simulink model "Multimedia_IP_traffic"  (R2021a)
settings: Solver=VariableStepAuto  StartTime=0.0  StopTime=10.0  RelTol=1e-3
settings Model: Creator=Ebenezer Sarpong  LastModifiedBy=Ebenezer Sarpong

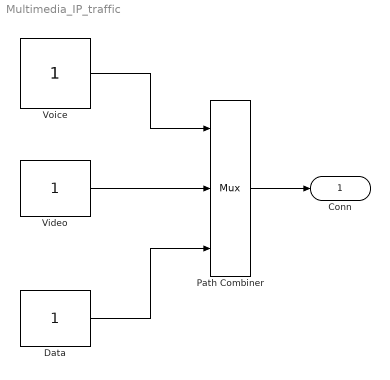
== system Multimedia_IP_traffic ==
  Data : Constant
  Path Combiner : Mux  Inputs=3
  Video : Constant
  Voice : Constant
  Conn : Outport
  wires:
  Voice/1 -> Path Combiner/1
  Data/1 -> Path Combiner/3
  Video/1 -> Path Combiner/2
  Path Combiner/1 -> Conn/1
